simulink model "PubIfCommonDMS_MDL"  (R2020b)
settings: Solver=FixedStepAuto  StartTime=0.0  StopTime=10.0  RelTol=1e-3
settings Model: DataDictionary=HWA_DDs.sldd  Creator=GW00180895  LastModifiedBy=GW00133806
settings ModelReferenceCC: ModelReferenceNumInstancesAllowed=Single

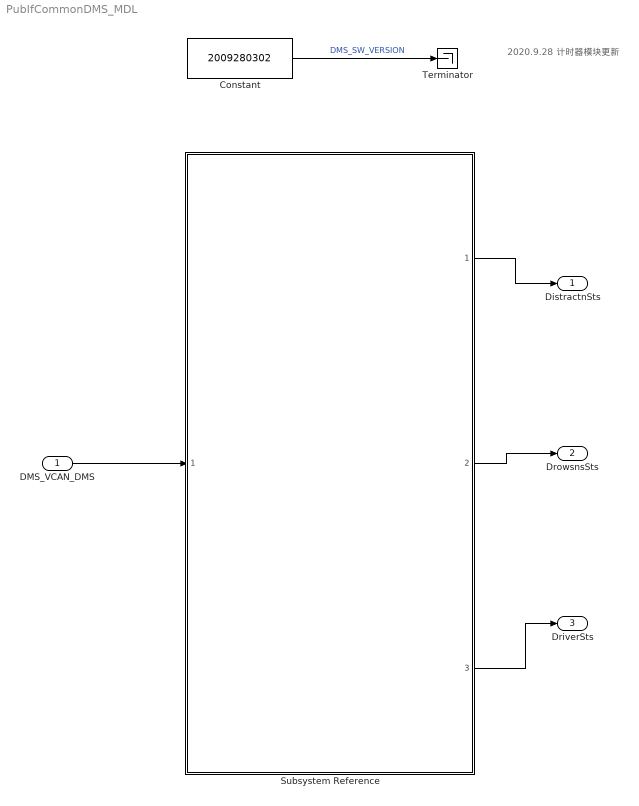
== system PubIfCommonDMS_MDL ==
  note: 2020.9.28
      | 计时器模块更新
  DMS_VCAN_DMS : Inport  OutDataTypeStr=Bus: VCAN_DMS_MSG_BUS  PortDimensions=1  BusOutputAsStruct=on
  Constant : Constant  Value=2009280302  OutDataTypeStr=uint32
  Subsystem Reference : Subsystem  ReferencedSubsystem=PvtSubSys_DMS
  Terminator : Terminator
  DistractnSts : Outport  OutDataTypeStr=uint8  PortDimensions=1  BusOutputAsStruct=on
  DrowsnsSts : Outport  Port=2  OutDataTypeStr=uint8  PortDimensions=1  BusOutputAsStruct=on
  DriverSts : Outport  Port=3  OutDataTypeStr=uint8  PortDimensions=1  BusOutputAsStruct=on
  wires:
  Constant/1 -> Terminator/1  "DMS_SW_VERSION"
  DMS_VCAN_DMS/1 -> Subsystem Reference/1
  Subsystem Reference/2 -> DrowsnsSts/1
  Subsystem Reference/1 -> DistractnSts/1
  Subsystem Reference/3 -> DriverSts/1
